simulink model "persistentExample_doubleDelays"  (R2017a)
settings: Solver=VariableStepAuto  StartTime=0.0  StopTime=10.0  RelTol=1e-3
settings Model: Creator=Dogan  LastModifiedBy=Dogan

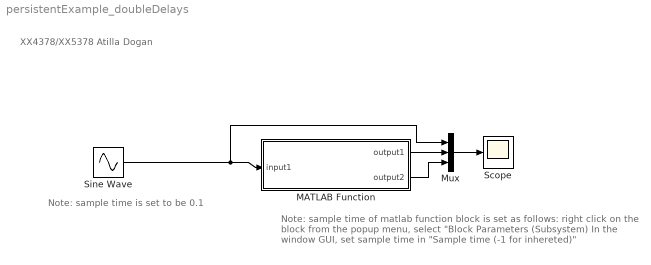
== system persistentExample_doubleDelays ==
  note: XX4378/XX5378
      | Atilla Dogan
  note: Note:
      | sample time of matlab function block is set as follows:
      | right click on the block
      | from the popup menu, select "Block Parameters (Subsystem)
      | In the window GUI, set sample time in "Sample time (-1 for inhereted)"
  note: Note: sample time is set to be 0.1
  MATLAB Function : MATLAB Function  TreatAsAtomicUnit=on  SystemSampleTime=.1
  Mux : Mux  Inputs=3
  Scope : Scope
  Sine Wave : Sin  Amplitude=10  SampleTime=0.1
  wires:
  Sine Wave/1 -> Mux/1, MATLAB Function/1(input1)
  Mux/1 -> Scope/1
  MATLAB Function/1(output1) -> Mux/2
  MATLAB Function/2(output2) -> Mux/3

== matlab function persistentExample_doubleDelays/MATLAB Function ==
  data: input1 input; output1 output; output2 output
function [output1,output2] = fcn(input1)
% An sample function to show how a persistent variable is declared and used
% in a function
% Atilla Dogan

persistent input1Pre input1PrePre

if isempty(input1Pre)
    input1Pre = 0; % if the initial condition is different than 0, replace the zero with the initial value
end

if isempty(input1PrePre)
    input1PrePre = 0; % if the initial condition is different than 0, replace the zero with the initial value
end

%% --------------------
% In this section (lines 9 to 16)
% you have access to the current value of the input (input1) and its previous value (input1Pre)

% as an example, if you want to output the previous value of the input
output1 = input1Pre;
output2 = input1PrePre;

%% --------------------
% These assignment should be the last lines in the function
input1PrePre = input1Pre;
input1Pre = input1;
return
